simulink model "sampleModel1416_3_sub_sub"  (R2023a)
settings: Solver=VariableStepAuto  StartTime=0.0  StopTime=10.0  RelTol=1e-3
libraries: simulink x2, hdlsllib x1
settings Model: Creator=user1  LastModifiedBy=user1

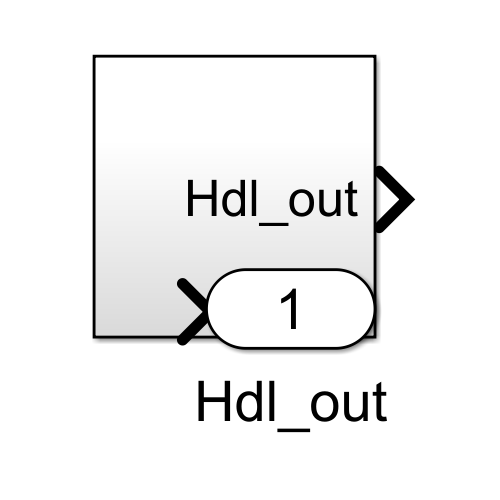
[thumbnail: Simulink's stored preview of the top-level diagram]
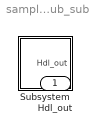
== system sampleModel1416_3_sub_sub ==
  Subsystem : Subsystem
  Hdl_out : Outport  OutDataTypeStr=uint8

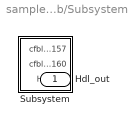
== system sampleModel1416_3_sub_sub/Subsystem ==
  Subsystem : Subsystem
  Hdl_out : Outport  OutDataTypeStr=uint8

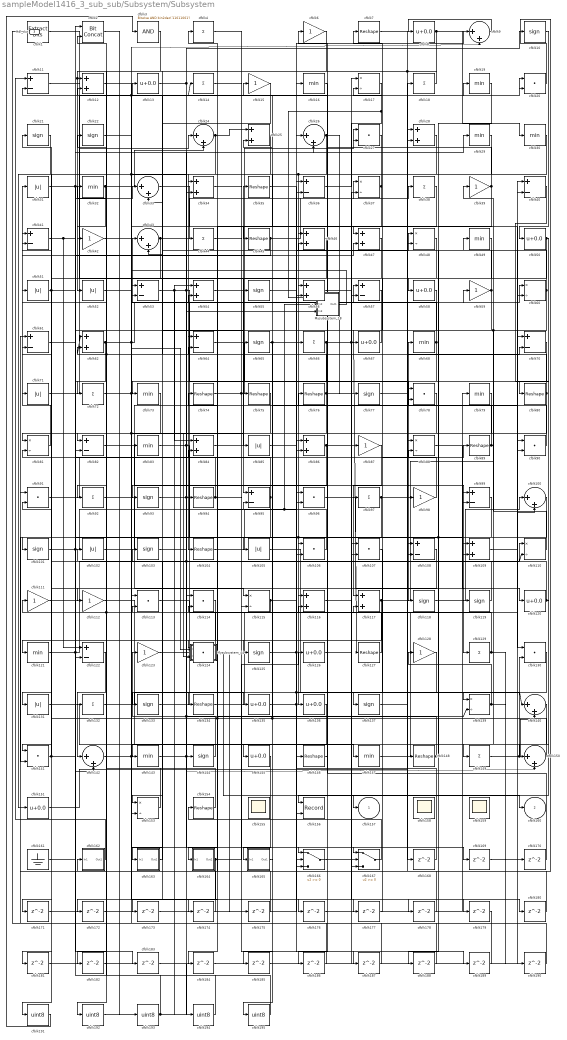
== system sampleModel1416_3_sub_sub/Subsystem/Subsystem ==
  Mysubsystem_18 : Subsystem  TreatAsAtomicUnit=on  RTWFcnName=Mysubsystem_18
      settings: RTWFcnNameOpts=User specified  RTWFileNameOpts=Use function name
  Mysubsystem_44 : Subsystem  TreatAsAtomicUnit=on  RTWFcnName=Mysubsystem_44
      settings: RTWFcnNameOpts=User specified  RTWFileNameOpts=Use function name
  cfblk1 : simulink/Logic and Bit Operations/Extract Bits  bitsToExtract=Upper half  numBits=8  bitIdxRange=[0 7]  outScalingMode=Preserve fixed-point scaling
      settings: LibrarySourceBlock=|
      | hdlsllib/Logic and Bit
      | Operations/Extract Bits
  cfblk{10,21..22,55,65,77,93,101,103,118..119,125,133,137,144} (15 alike) : Signum
  cfblk{9,24,26,33,43,100,140,142,150} (9 alike) : Sum  Inputs=|++  OutDataTypeStr=uint8
  cfblk{31,51..52,71,85,102,105,131} (8 alike) : Abs  OutDataTypeStr=uint8  SaturateOnIntegerOverflow=off
  cfblk{7,35,45,74..76,80,89,94,104,127,134,146,148,154} (15 alike) : Reshape
  cfblk{20,27,78,90..91,96,106..107,113..114,124,130,141} (13 alike) : DotProduct  OutDataTypeStr=uint8
  cfblk{11,36,40..41,53,57,61,64,70,82,95,99,108,122} (14 alike) : Sum  Inputs=+-  OutDataTypeStr=uint8
  cfblk{12,25,28,34,46..47,54,56,62,84,86,109,116..117} (14 alike) : Sum  OutDataTypeStr=uint8
  cfblk{17,37,48,60,81,88,110,115,139,153} (10 alike) : Product  Inputs=*/  OutDataTypeStr=uint8  RndMeth=Zero  SaturateOnIntegerOverflow=on
  cfblk{6,15,39,42,59,87,98,111..112,123,128} (11 alike) : Gain  OutDataTypeStr=uint8
  cfblk{8,13,50,58,67,120,126,135..136,145,151} (11 alike) : Bias  Bias=0.0  SaturateOnIntegerOverflow=off
  cfblk{16,19,29..30,32,49,68,73,79,83,121,143,147} (13 alike) : MinMax  OutDataTypeStr=uint8
  cfblk{4,14,18,38,44,66,72,92,97,129,132,149} (12 alike) : Sum  Inputs=+  OutDataTypeStr=uint8
  cfblk155 : Scope
      settings: Floating=on
  cfblk156 : Record  FileSettingsInternal="{\"entries\":[{\"content\":{\"excelSettings\":{\"content\":{},\"type\":\"Streamout.ExcelSettings\"}},\"type\":\"Streamout.FileSettingStorage\",\"uuid\":\"\"}],\"packageUris\":[\"http:\\/\\/schema.mathworks.com\\/mf0\\/streamout_blocks\\/R2020a\"],\"version\":\"1.0\"}"  Layout=[1 1]  SignalsInternal="{\"entries\":[{\"content\":{\"signals\":[{\"content\":{\"blockPath\":[],\"dimensions\":[1],\"domain\":\"\",\"lineColor\":\"#a2142f\",\"plots\":[1],\"port\":1,\"signalID\":14164,\"signalName\":\"cfblk40\"},\"type\":\"RecordBlkView.Signal\",\"uuid\":\"\"},{\"content\":{\"blockPath\":[],\"dimensions\":[1],\"domain\":\"\",\"lineColor\":\"#139fff\",\"plots\":[1],\"port\":2,\"signalID\":14167,\"signalName\":\"cfblk112\"},\"type\":\"RecordBlkView.Signal\",\"uuid\":\"\"}]},\"type\":\"RecordBlkView.InputSignals\",\"uuid\":\"\"}],\"packageUris\":[\"http:\\/\\/schema.mathworks.com\\/mf0\\/streamout_blocks\\/R2020a\"],\"version\":\"1.0\"}"  VisualizationBindings="{\"xyplotplugin\":{\"info\":[{\"series\":[{\"bindingParametersList\":[{\"parameter\":\"X-Axis\",\"signalID\":14164,\"signalName\":\"cfblk40\"},{\"parameter\":\"Y-Axis\",\"signalID\":14167,\"signalName\":\"cfblk112\"}],\"seriesID\":22364}],\"subplotID\":1}]}}"  CompatibilityTag=XY  st=-1
  cfblk158 : Scope
      settings: Floating=on
  cfblk159 : Scope
      settings: Floating=on
  cfblk161 : Ground
  cfblk162 : Subsystem
      settings: LibrarySourceBlock=|
      | hdlsllib/Ports &
      | Subsystems/Subsystem
  cfblk163 : Subsystem
      settings: LibrarySourceBlock=|
      | hdlsllib/Ports &
      | Subsystems/Subsystem
  cfblk164 : Subsystem
      settings: LibrarySourceBlock=|
      | hdlsllib/Ports &
      | Subsystems/Subsystem
  cfblk165 : Subsystem
      settings: LibrarySourceBlock=|
      | hdlsllib/Ports &
      | Subsystems/Subsystem
  cfblk166 : Switch  OutDataTypeStr=uint8  SaturateOnIntegerOverflow=off  InputSameDT=off
  cfblk167 : Switch  OutDataTypeStr=uint8  SaturateOnIntegerOverflow=off  InputSameDT=off
  cfblk{168..190} (23 alike) : Delay  SampleTime=1
  cfblk{191..195} (5 alike) : DataTypeConversion  OutDataTypeStr=uint8  SaturateOnIntegerOverflow=off  RndMeth=Floor
  cfblk2 : hdlsllib/Logic and Bit Operations/Bit Concat  numInputs=2
  cfblk3 : simulink/Logic and Bit Operations/Bitwise Operator  logicop=AND  UseBitMask=on  BitMask=bin2dec('11011001')  BitMaskRealWorld=Stored Integer
      settings: LibrarySourceBlock=|
      | hdlsllib/Logic and Bit
      | Operations/Bitwise
      | Operator
  cfblk157 : Outport  OutDataTypeStr=uint8  VectorParamsAs1DForOutWhenUnconnected=off
  cfblk160 : Outport  Port=2  OutDataTypeStr=uint8  VectorParamsAs1DForOutWhenUnconnected=off
  Hdl_out : Outport  Port=3  OutDataTypeStr=uint8
  wires:
  Mysubsystem_44/1(cfblk157) -> cfblk157/1
  cfblk78/1 -> Mysubsystem_44/2(In2)
  Mysubsystem_18/1(Out1) -> Mysubsystem_44/1(In1)
  cfblk195/1 -> cfblk2/2
  cfblk165/1(Out1) -> cfblk195/1
  cfblk194/1 -> cfblk2/1
  cfblk183/1 -> cfblk194/1
  cfblk193/1 -> cfblk22/1, cfblk54/1
  cfblk192/1 -> cfblk94/1, cfblk44/1
  cfblk191/1 -> cfblk3/1
  cfblk28/1 -> cfblk191/1
  cfblk190/1 -> cfblk53/1
  cfblk189/1 -> cfblk167/2
  cfblk188/1 -> cfblk107/1
  cfblk187/1 -> cfblk62/2
  cfblk4/1 -> cfblk187/1
  cfblk186/1 -> cfblk61/1
  cfblk38/1 -> cfblk186/1
  cfblk185/1 -> cfblk60/2
  cfblk184/1 -> cfblk70/1
  cfblk58/1 -> cfblk184/1
  cfblk182/1 -> cfblk57/2
  cfblk25/1 -> cfblk182/1
  cfblk181/1 -> cfblk100/2
  cfblk180/1 -> cfblk54/2
  cfblk14/1 -> cfblk180/1
  cfblk179/1 -> cfblk1/1
  cfblk56/1 -> cfblk179/1
  cfblk178/1 -> cfblk88/1
  cfblk52/1 -> cfblk178/1
  cfblk177/1 -> cfblk17/2
  cfblk34/1 -> cfblk177/1
  cfblk176/1 -> cfblk99/1
  cfblk175/1 -> cfblk84/2
  cfblk174/1 -> cfblk91/1
  cfblk128/1 -> cfblk174/1
  cfblk173/1 -> cfblk86/2
  cfblk136/1 -> cfblk173/1
  cfblk172/1 -> cfblk113/1
  cfblk171/1 -> cfblk36/2
  cfblk108/1 -> cfblk171/1
  cfblk170/1 -> cfblk116/2
  cfblk169/1 -> cfblk90/1
  cfblk168/1 -> cfblk96/1
  cfblk7/1 -> cfblk168/1
  cfblk83/1 -> cfblk106/1, cfblk26/2
  cfblk111/1 -> cfblk110/1
  cfblk79/1 -> cfblk82/2
  cfblk149/1 -> cfblk130/2, cfblk140/2
  cfblk44/1 -> cfblk97/1
  cfblk95/1 -> cfblk141/2, cfblk81/2
  cfblk35/1 -> cfblk167/1
  cfblk93/1 -> cfblk98/1
  cfblk72/1 -> cfblk9/2, cfblk14/1, cfblk85/1
  cfblk137/1 -> cfblk70/2
  cfblk121/1 -> cfblk26/1, cfblk33/1
  cfblk29/1 -> cfblk45/1
  cfblk48/1 -> cfblk67/1
  cfblk119/1 -> cfblk91/2
  cfblk116/1 -> cfblk60/1
  cfblk125/1 -> cfblk146/1, cfblk140/1, cfblk48/1
  cfblk163/1(Out1) -> cfblk103/1
  cfblk37/1 -> cfblk34/1, cfblk134/1
  cfblk47/1 -> cfblk92/1
  cfblk89/1 -> cfblk109/1, cfblk55/1
  cfblk140/1 -> cfblk145/1
  cfblk51/1 -> cfblk101/1, cfblk105/1
  cfblk142/1 -> cfblk19/1, cfblk166/3
  cfblk70/1 -> cfblk133/1
  cfblk12/1 -> cfblk34/2, cfblk176/1
  cfblk120/1 -> cfblk46/2, cfblk150/1
  cfblk1/1 -> cfblk96/2
  cfblk75/1 -> cfblk124/1
  cfblk161/1 -> cfblk142/2
  cfblk60/1 -> cfblk149/1, cfblk188/1, cfblk6/1
  cfblk33/1 -> cfblk130/1
  cfblk109/1 -> cfblk40/2
  cfblk46/1 -> cfblk72/1
  cfblk50/1 -> cfblk75/1, cfblk80/1
  cfblk80/1 -> cfblk131/1, cfblk33/2
  cfblk113/1 -> cfblk117/2
  cfblk97/1 -> cfblk148/1, cfblk124/2
  cfblk85/1 -> cfblk27/2
  cfblk144/1 -> cfblk123/1
  cfblk73/1 -> cfblk141/1
  cfblk132/1 -> cfblk135/1
  cfblk22/1 -> cfblk83/1
  cfblk164/1(Out1) -> cfblk126/1, cfblk172/1
  cfblk145/1 -> cfblk165/1(In1)
  cfblk8/1 -> cfblk28/2, cfblk112/1, cfblk30/1
  cfblk112/1 -> cfblk156/2
  cfblk96/1 -> cfblk119/1
  cfblk17/1 -> Mysubsystem_18/1(In1), cfblk107/2
  cfblk20/1 -> cfblk162/1(In1)
  cfblk16/1 -> cfblk46/1
  cfblk57/1 -> cfblk53/2
  cfblk129/1 -> cfblk113/2, cfblk170/1
  cfblk166/1 -> cfblk87/1
  cfblk134/1 -> cfblk16/1
  cfblk64/1 -> cfblk78/2
  cfblk24/1 -> cfblk25/1, cfblk181/1
  cfblk130/1 -> cfblk163/1(In1)
  cfblk146/1 -> cfblk76/1
  cfblk77/1 -> cfblk28/1
  cfblk84/1 -> cfblk35/1
  cfblk62/1 -> cfblk36/1, cfblk59/1, cfblk122/2
  cfblk162/1(Out1) -> cfblk11/1
  cfblk115/1 -> cfblk20/2, cfblk114/2
  cfblk135/1 -> cfblk9/1, cfblk189/1
  cfblk153/1 -> cfblk102/1
  cfblk82/1 -> cfblk129/1
  cfblk104/1 -> cfblk56/2
  cfblk100/1 -> cfblk116/1, cfblk125/1
  cfblk86/1 -> cfblk93/1, cfblk99/2
  cfblk41/1 -> cfblk122/1, cfblk183/1
  cfblk124/1 -> cfblk71/1, cfblk12/2, cfblk175/1
  cfblk76/1 -> cfblk132/1, cfblk153/2, cfblk37/2, cfblk32/1
  cfblk55/1 -> cfblk86/1
  cfblk15/1 -> cfblk43/2
  cfblk74/1 -> cfblk27/1, cfblk108/2
  cfblk87/1 -> cfblk117/1
  cfblk30/1 -> cfblk56/1, cfblk115/2
  cfblk2/1 -> cfblk193/1
  cfblk94/1 -> cfblk166/1, cfblk21/1
  cfblk39/1 -> cfblk108/1, cfblk11/2
  cfblk167/1 -> cfblk154/1
  cfblk133/1 -> cfblk90/2
  cfblk102/1 -> cfblk40/1
  cfblk42/1 -> cfblk47/1
  cfblk101/1 -> cfblk95/2, cfblk47/2
  cfblk61/1 -> cfblk29/1
  cfblk151/1 -> cfblk18/1
  cfblk32/1 -> cfblk24/2, cfblk42/1
  cfblk88/1 -> cfblk120/1
  cfblk98/1 -> cfblk7/1
  cfblk150/1 -> cfblk64/2, cfblk61/2, cfblk15/1
  cfblk106/1 -> cfblk4/1, Mysubsystem_18/2(In2)
  cfblk141/1 -> cfblk111/1, cfblk88/2
  cfblk3/1 -> cfblk192/1
  cfblk54/1 -> cfblk95/1
  cfblk126/1 -> cfblk160/1
  cfblk143/1 -> Mysubsystem_18/3(In3), cfblk139/2, cfblk144/1, cfblk150/2
  cfblk139/1 -> cfblk48/2, cfblk190/1
  cfblk6/1 -> cfblk73/1
  cfblk59/1 -> cfblk153/1, cfblk13/1
  cfblk118/1 -> cfblk100/1
  cfblk107/1 -> cfblk137/1
  cfblk65/1 -> cfblk66/1, cfblk185/1
  cfblk21/1 -> cfblk151/1
  cfblk127/1 -> cfblk41/1
  cfblk122/1 -> cfblk142/1
  cfblk11/1 -> cfblk64/1
  cfblk49/1 -> cfblk82/1
  cfblk114/1 -> cfblk121/1
  cfblk40/1 -> cfblk156/1
  cfblk13/1 -> cfblk114/1, cfblk10/1
  cfblk154/1 -> cfblk62/1, cfblk51/1
  cfblk53/1 -> cfblk78/1, cfblk167/3, cfblk84/1
  cfblk81/1 -> cfblk31/1
  cfblk148/1 -> cfblk74/1, cfblk128/1
  cfblk147/1 -> cfblk79/1
  cfblk131/1 -> cfblk147/1
  cfblk90/1 -> cfblk68/1
  cfblk19/1 -> cfblk58/1
  cfblk26/1 -> cfblk104/1, cfblk77/1
  cfblk123/1 -> cfblk57/1
  cfblk9/1 -> cfblk8/1
  cfblk67/1 -> cfblk43/1
  cfblk105/1 -> cfblk139/1
  cfblk31/1 -> cfblk24/1, cfblk65/1
  cfblk18/1 -> cfblk52/1, cfblk12/1
  cfblk36/1 -> cfblk17/1
  cfblk66/1 -> cfblk127/1, cfblk109/2, cfblk166/2
  cfblk43/1 -> cfblk37/1, cfblk81/1
  cfblk103/1 -> cfblk110/2, cfblk169/1
  cfblk10/1 -> cfblk50/1
  cfblk110/1 -> cfblk49/1
  cfblk27/1 -> cfblk136/1
  cfblk99/1 -> cfblk143/1, cfblk106/2
  cfblk68/1 -> cfblk118/1, cfblk25/2
  cfblk45/1 -> cfblk38/1, cfblk41/2
  cfblk92/1 -> cfblk115/1
  cfblk71/1 -> cfblk20/1
  cfblk117/1 -> cfblk39/1, cfblk164/1(In1)
  cfblk91/1 -> cfblk89/1

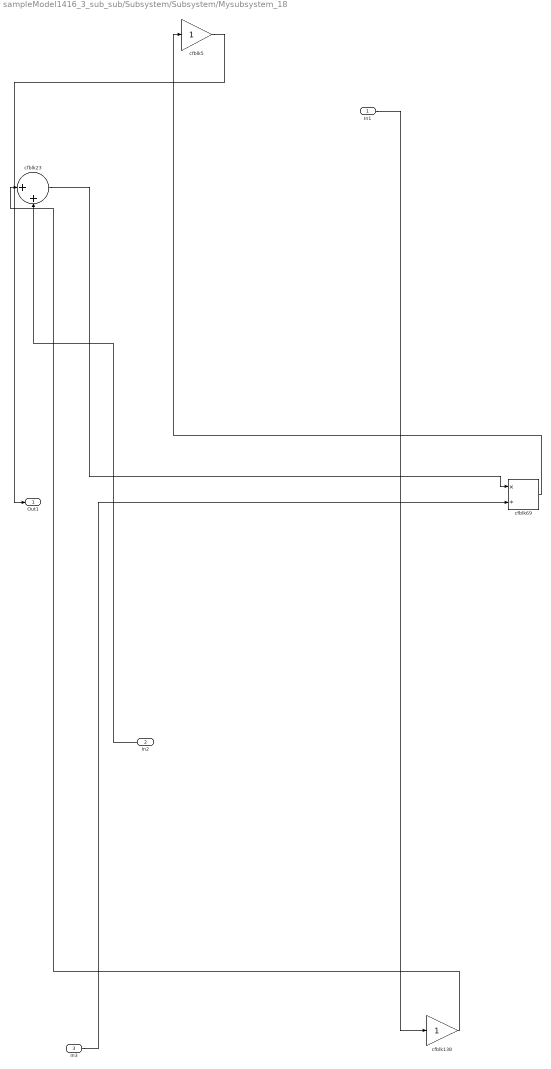
== system sampleModel1416_3_sub_sub/Subsystem/Subsystem/Mysubsystem_18 ==
  In1 : Inport
  In2 : Inport  Port=2
  In3 : Inport  Port=3
  cfblk138 : Gain
  cfblk23 : Sum  Inputs=|++
  cfblk5 : Gain
  cfblk69 : Product  Inputs=*/  RndMeth=Zero  SaturateOnIntegerOverflow=on
  Out1 : Outport
  wires:
  cfblk138/1 -> cfblk23/1
  cfblk23/1 -> cfblk69/1
  In3/1 -> cfblk69/2
  cfblk69/1 -> cfblk5/1
  In2/1 -> cfblk23/2
  In1/1 -> cfblk138/1
  cfblk5/1 -> Out1/1

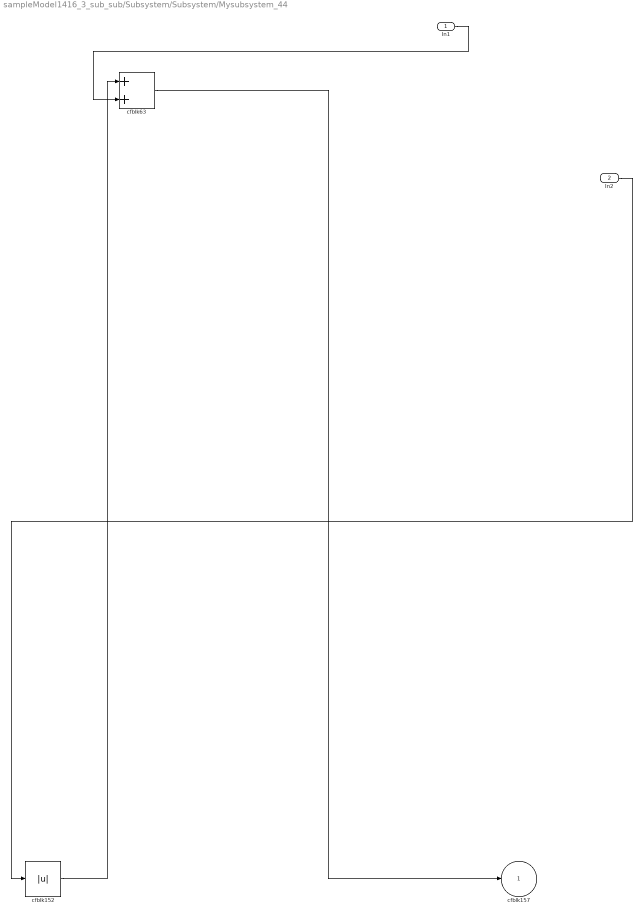
== system sampleModel1416_3_sub_sub/Subsystem/Subsystem/Mysubsystem_44 ==
  In1 : Inport
  In2 : Inport  Port=2
  cfblk152 : Abs  SaturateOnIntegerOverflow=off
  cfblk63 : Sum
  cfblk157 : Outport  VectorParamsAs1DForOutWhenUnconnected=off
  wires:
  cfblk152/1 -> cfblk63/1
  cfblk63/1 -> cfblk157/1
  In1/1 -> cfblk63/2
  In2/1 -> cfblk152/1

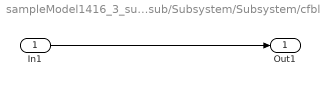
== system sampleModel1416_3_sub_sub/Subsystem/Subsystem/cfblk162 ==
  In1 : Inport
  Out1 : Outport
  wires:
  In1/1 -> Out1/1

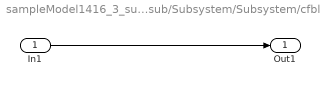
== system sampleModel1416_3_sub_sub/Subsystem/Subsystem/cfblk163 ==
  In1 : Inport
  Out1 : Outport
  wires:
  In1/1 -> Out1/1

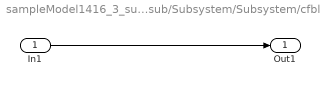
== system sampleModel1416_3_sub_sub/Subsystem/Subsystem/cfblk164 ==
  In1 : Inport
  Out1 : Outport
  wires:
  In1/1 -> Out1/1

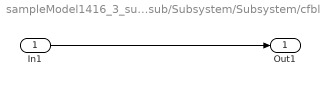
== system sampleModel1416_3_sub_sub/Subsystem/Subsystem/cfblk165 ==
  In1 : Inport
  Out1 : Outport
  wires:
  In1/1 -> Out1/1
